simulink model "FullModel"  (R2021a)
settings: Solver=VariableStepAuto  StartTime=0.0  StopTime=5  MaxStep=0.01  RelTol=1e-3
values from neighbouring files (symbols this model uses):
  Tau_hm = 1e-3    (= 0.001)    [Data.m]
  Tau_tm = 1e-3    (= 0.001)    [Data.m]
  Thm_max = 2.0e4    (= 20000)    [Data.m]
  Ttm_max = 3.0e3    (= 3000)    [Data.m]
settings Model: Creator=jpss8  LastModifiedBy=jpss8

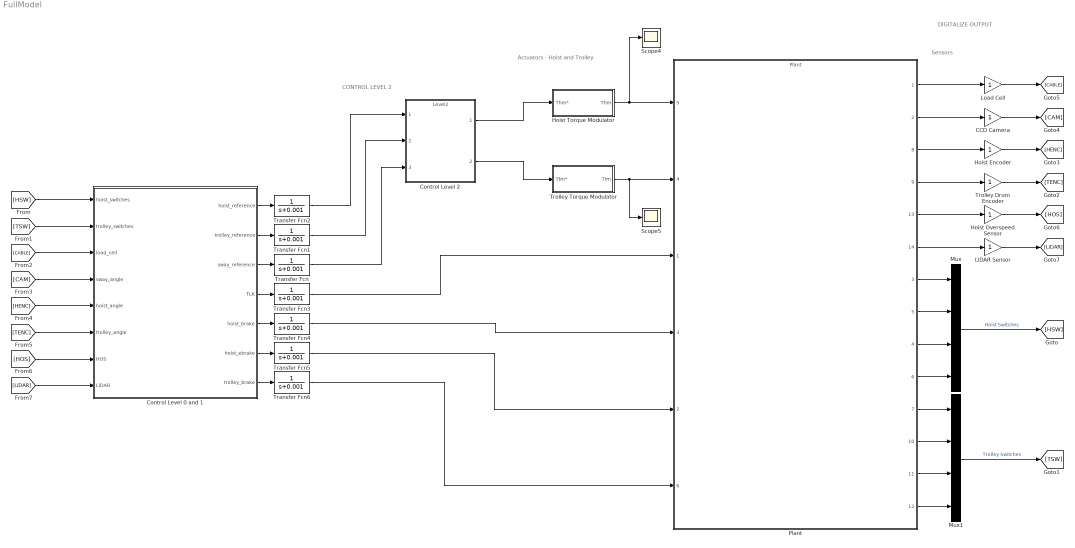
== system FullModel ==
  note: DIGITALIZE OUTPUT
  note: CONTROL LEVEL 2
  note: Sensors
  note: Actuators - Hoist and Trolley
  CCD Camera : Gain
  Control Level 0 and 1 : Subsystem
  Control Level 2 : ModelReference  ModelNameDialog=Level2.slx  SimulationMode=Normal  ModelReferenceVersion=1.6
  Hoist Encoder : Gain
  Hoist Overspeed Sensor : Gain
  Hoist Torque Modulator : Subsystem
  LiDAR Sensor : Gain
  Load Cell : Gain
  Mux : Mux
  Mux1 : Mux
  Plant : ModelReference  ModelNameDialog=Plant.slx  SimulationMode=Normal  ModelReferenceVersion=1.105
      settings: PortSchema="{\"entries\":[{\"content\":{\"sides\":[{\"content\":{\"connectorIds\":[\"In5\",\"In4\",\"In1\",\"In3\",\"In2\",\"In6\"]},\"type\":\"ConnectorPlacement.EquallySpacedRectSide\",\"uuid\":\"21bb6514-2ae1-4e91-8ba8-0048b23f5eee\"},{\"content\":{\"connectorIds\":[\"Out1\",\"Out2\",\"Out8\",\"Out9\",\"Out13\",\"Out14\",\"Out3\",\"Out5\",\"Out4\",\"Out6\",\"Out7\",\"Out10\",\"Out11\",\"Out12\"],\"side\":\"RIGHT\"},\"type\":\"ConnectorPlacement.EquallySpacedRectSide\",\"uuid\":\"76781d7b-468f-4fab-8408-33b7b044b816\"},{\"content\":{\"connectorIds\":[],\"side\":\"TOP\"},\"type\":\"ConnectorPlacement.EquallySpacedRectSide\",\"uuid\":\"b4764fd0-dcaa-4ab7-bf15-0e4691eece23\"}]},\"type\":\"ConnectorPlacement.EquallySpacedConnector\",\"uuid\":\"81ec6fbc-127c-46f8-9807-91263d11131f\"}],\"packageUris\":[\"http://schema.mathworks.com/mf0/Connector/R2020b\"],\"version\":\"1.0\"}"
  Scope4 : Scope
  Scope5 : Scope
  Transfer Fcn{,1..6} (7 alike) : TransferFcn  Denominator=[1 0.001]
  Trolley Drum Encoder : Gain
  Trolley Torque Modulator : Subsystem
  wires:
  Trolley Torque Modulator/1(Ttm) -> Scope5/1, Plant/4
  Hoist Torque Modulator/1(Thm) -> Plant/5, Scope4/1
  Plant/1 -> Load Cell/1
  Plant/2 -> CCD Camera/1
  Plant/8 -> Hoist Encoder/1
  Plant/9 -> Trolley Drum Encoder/1
  Plant/3 -> Mux/1
  Plant/5 -> Mux/2
  Plant/4 -> Mux/3
  Plant/6 -> Mux/4
  Plant/7 -> Mux1/1
  Plant/10 -> Mux1/2
  Plant/11 -> Mux1/3
  Plant/12 -> Mux1/4
  Mux/1 -> [HSW]  "Hoist Switches"
  Mux1/1 -> [TSW]  "Trolley Switches"
  Control Level 2/1 -> Hoist Torque Modulator/1(Thm*)
  Control Level 2/2 -> Trolley Torque Modulator/1(Ttm*)
  Trolley Drum Encoder/1 -> [TENC]
  Hoist Encoder/1 -> [HENC]
  Load Cell/1 -> [CABLE]
  CCD Camera/1 -> [CAM]
  Plant/13 -> Hoist Overspeed Sensor/1
  Hoist Overspeed Sensor/1 -> [HOS]
  Transfer Fcn3/1 -> Plant/1
  Transfer Fcn4/1 -> Plant/3
  Transfer Fcn5/1 -> Plant/2
  Transfer Fcn6/1 -> Plant/6
  Transfer Fcn2/1 -> Control Level 2/1
  Transfer Fcn/1 -> Control Level 2/3
  Transfer Fcn1/1 -> Control Level 2/2
  [HSW] -> Control Level 0 and 1/1(hoist_switches)
  [TSW] -> Control Level 0 and 1/2(trolley_switches)
  [CABLE] -> Control Level 0 and 1/3(load_cell)
  [CAM] -> Control Level 0 and 1/4(sway_angle)
  [HENC] -> Control Level 0 and 1/5(hoist_angle)
  [TENC] -> Control Level 0 and 1/6(trolley_angle)
  [HOS] -> Control Level 0 and 1/7(HOS)
  Control Level 0 and 1/1(hoist_reference) -> Transfer Fcn2/1
  Control Level 0 and 1/2(trolley_reference) -> Transfer Fcn1/1
  Control Level 0 and 1/3(sway_reference) -> Transfer Fcn/1
  Control Level 0 and 1/4(TLK) -> Transfer Fcn3/1
  Control Level 0 and 1/5(hoist_brake) -> Transfer Fcn4/1
  Control Level 0 and 1/6(hoist_ebrake) -> Transfer Fcn5/1
  Control Level 0 and 1/7(trolley_brake) -> Transfer Fcn6/1
  LiDAR Sensor/1 -> [LiDAR]
  Plant/14 -> LiDAR Sensor/1
  [LiDAR] -> Control Level 0 and 1/8(LiDAR)

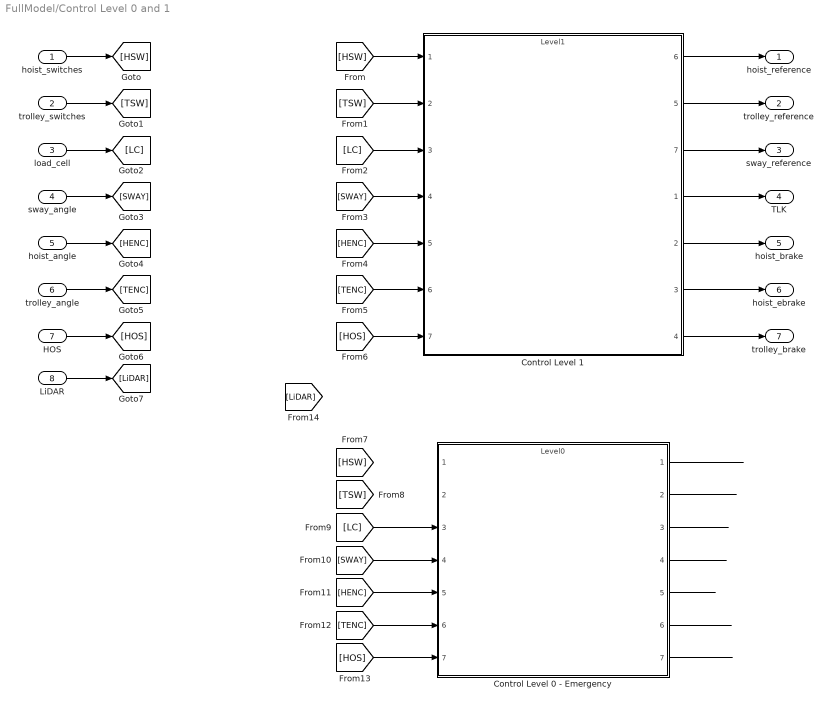
== system FullModel/Control Level 0 and 1 ==
  hoist_switches : Inport
  trolley_switches : Inport  Port=2
  load_cell : Inport  Port=3
  sway_angle : Inport  Port=4
  hoist_angle : Inport  Port=5
  trolley_angle : Inport  Port=6
  HOS : Inport  Port=7
  LiDAR : Inport  Port=8
  Control Level 0 - Emergency : ModelReference  ModelNameDialog=Level0.slx  SimulationMode=Normal  ModelReferenceVersion=1.5
  Control Level 1 : ModelReference  ModelNameDialog=Level1.slx  SimulationMode=Normal  ModelReferenceVersion=1.9
      settings: PortSchema="{\"entries\":[{\"content\":{\"sides\":[{\"content\":{\"connectorIds\":[\"In1\",\"In2\",\"In3\",\"In4\",\"In5\",\"In6\",\"In7\"]},\"type\":\"ConnectorPlacement.EquallySpacedRectSide\",\"uuid\":\"c895f490-3284-4b93-bf43-b0d895c4aa94\"},{\"content\":{\"connectorIds\":[\"Out6\",\"Out5\",\"Out7\",\"Out1\",\"Out2\",\"Out3\",\"Out4\"],\"side\":\"RIGHT\"},\"type\":\"ConnectorPlacement.EquallySpacedRectSide\",\"uuid\":\"9f33a06e-257b-4f07-9596-dd3a7917b54b\"},{\"content\":{\"connectorIds\":[],\"side\":\"TOP\"},\"type\":\"ConnectorPlacement.EquallySpacedRectSide\",\"uuid\":\"d9489eda-7aa0-457f-99be-386f84b0da79\"}]},\"type\":\"ConnectorPlacement.EquallySpacedConnector\",\"uuid\":\"c8749ef1-ab8d-464e-907f-fbff5a657293\"}],\"packageUris\":[\"http://schema.mathworks.com/mf0/Connector/R2020b\"],\"version\":\"1.0\"}"
  hoist_reference : Outport
  trolley_reference : Outport  Port=2
  sway_reference : Outport  Port=3
  TLK : Outport  Port=4
  hoist_brake : Outport  Port=5
  hoist_ebrake : Outport  Port=6
  trolley_brake : Outport  Port=7
  wires:
  Control Level 1/7 -> sway_reference/1
  Control Level 1/4 -> trolley_brake/1
  Control Level 1/2 -> hoist_brake/1
  Control Level 1/6 -> hoist_reference/1
  Control Level 1/3 -> hoist_ebrake/1
  Control Level 1/1 -> TLK/1
  Control Level 1/5 -> trolley_reference/1
  hoist_switches/1 -> [HSW]
  trolley_switches/1 -> [TSW]
  load_cell/1 -> [LC]
  sway_angle/1 -> [SWAY]
  hoist_angle/1 -> [HENC]
  trolley_angle/1 -> [TENC]
  HOS/1 -> [HOS]
  [HSW] -> Control Level 1/1
  [TSW] -> Control Level 1/2
  [HOS] -> Control Level 1/7
  [TENC] -> Control Level 1/6
  [HENC] -> Control Level 1/5
  [SWAY] -> Control Level 1/4
  [LC] -> Control Level 1/3
  [HOS] -> Control Level 0 - Emergency/7
  [SWAY] -> Control Level 0 - Emergency/4
  [TENC] -> Control Level 0 - Emergency/6
  [HENC] -> Control Level 0 - Emergency/5
  [LC] -> Control Level 0 - Emergency/3
  Control Level 0 - Emergency/1 -> ?
  Control Level 0 - Emergency/2 -> ?
  Control Level 0 - Emergency/3 -> ?
  Control Level 0 - Emergency/4 -> ?
  Control Level 0 - Emergency/5 -> ?
  Control Level 0 - Emergency/6 -> ?
  Control Level 0 - Emergency/7 -> ?
  LiDAR/1 -> [LiDAR]

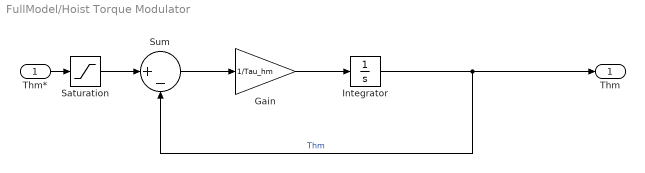
== system FullModel/Hoist Torque Modulator ==
  Thm* : Inport
  Gain : Gain  Gain=1/Tau_hm
  Integrator : Integrator
  Saturation : Saturate  UpperLimit=Thm_max  LowerLimit=-Thm_max
  Sum : Sum  Inputs=|+-
  Thm : Outport
  wires:
  Thm*/1 -> Saturation/1
  Integrator/1 -> Sum/2, Thm/1  "Thm"
  Sum/1 -> Gain/1
  Gain/1 -> Integrator/1
  Saturation/1 -> Sum/1

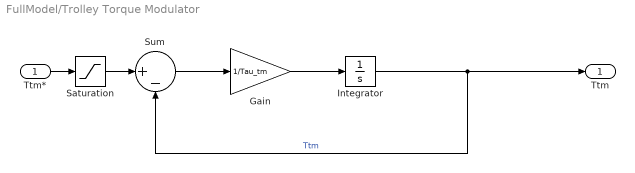
== system FullModel/Trolley Torque Modulator ==
  Ttm* : Inport
  Gain : Gain  Gain=1/Tau_tm
  Integrator : Integrator
  Saturation : Saturate  UpperLimit=Ttm_max  LowerLimit=-Ttm_max
  Sum : Sum  Inputs=|+-
  Ttm : Outport
  wires:
  Ttm*/1 -> Saturation/1
  Gain/1 -> Integrator/1
  Sum/1 -> Gain/1
  Integrator/1 -> Ttm/1, Sum/2  "Ttm"
  Saturation/1 -> Sum/1
